simulink model "fixed_point_filter_converter"  (R2020a)
settings: Solver=FixedStepAuto  StartTime=0  StopTime=Inf  RelTol=1e-3
model workspace (MAT data in the model file):
  a = 0
settings Model: MinMaxOverflowLogging=MinMaxAndOverflow  FPTRunName=EmbeddedRun  FPTShortcutValueString='{{},{''BaselineRun_3'',1,1,1,''BaselineRun_3'','''',{},''M'',''D'',''''},{''EmbeddedRun'',1,1,1,''EmbeddedRun'','''',{},''M'','''',''''},{''BaselineRun'',1,1,1,''BaselineRun'','''',{},''M'',''D'',''''},{''BaselineRun_2'',1,1,1,''BaselineRun_2'','''',{},''M'',''D'',''''},{''EmbeddedRun_2'',1,1,1,''EmbeddedRun_2'','''',{},''M'','''',''''},{''BaselineRun_4'',1,1,1,''BaselineRun_4'','''',{},''M'',''D'',''''},{''BaselineRun_7'',1,1,1,''BaselineRun_7'','''',{},''M'',''D'',''''}}'  Creator=sbuccelli  LastModifiedBy=diflo
settings DataIOCC: SaveOutput=off  SaveTime=off
settings OptimizationCC: BlockReduction=off  ConditionallyExecuteInputs=off  DefaultParameterBehavior=Inlined
settings DebuggingCC: SignalRangeChecking=error  AlgebraicLoopMsg=error  SingleTaskRateTransMsg=error  IntegerOverflowMsg=none  ParameterDowncastMsg=none  ParameterOverflowMsg=none  ParameterPrecisionLossMsg=none  IntegerSaturationMsg=none
settings HardwareCC: ProdBitPerPointer=32  ProdBitPerSizeT=32  ProdBitPerPtrDiffT=32  ProdLargestAtomicFloat=None  ProdIntDivRoundTo=Undefined  ProdEndianess=Unspecified  ProdWordSize=32  ProdHWDeviceType=ASIC/FPGA->ASIC/FPGA  TargetBitPerPointer=64  TargetBitPerSizeT=64  TargetBitPerPtrDiffT=64  TargetLongLongMode=on  TargetIntDivRoundTo=Zero  TargetEndianess=LittleEndian  TargetWordSize=64  TargetHWDeviceType=Custom Processor->MATLAB Host Computer  ProdEqTarget=off

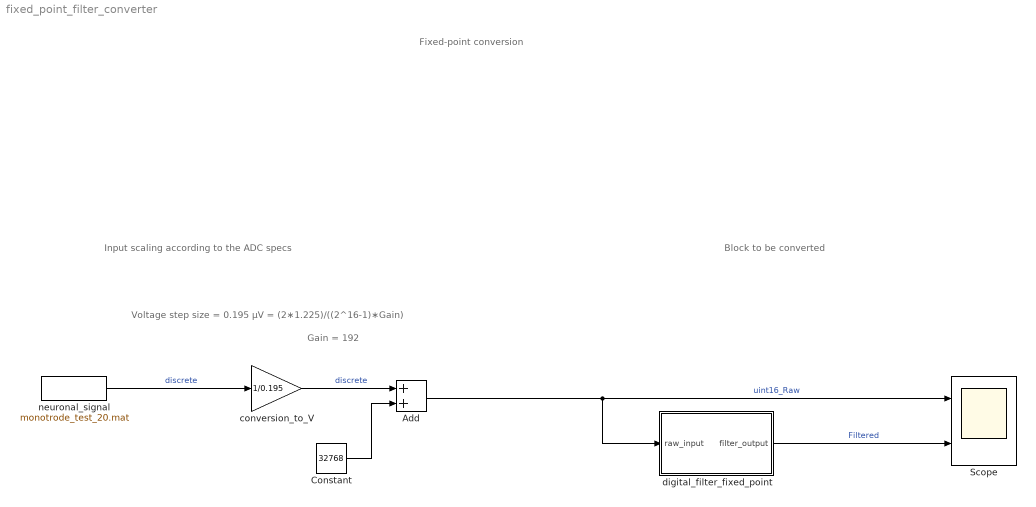
== system fixed_point_filter_converter ==
  note: Input scaling according to the ADC specs
  note: Gain = 192
  note: Voltage step size = 0.195 µV = (2∗1.225)/((2^16-1)∗Gain)
  note: Fixed-point conversion
  note: Block to be converted
  Add : Sum  OutDataTypeStr=uint16
  Constant : Constant  Value=32768  OutDataTypeStr=uint16  SampleTime=-1
  Scope : Scope  NumInputPorts=2
  conversion_to_V : Gain  Gain=1/0.195
  digital_filter_fixed_point : Subsystem
  neuronal_signal : FromFile  FileName=monotrode_test_20.mat  SampleTime=1/30000
  wires:
  neuronal_signal/1 -> conversion_to_V/1  "discrete"
  conversion_to_V/1 -> Add/1  "discrete"
  Constant/1 -> Add/2
  Add/1 -> digital_filter_fixed_point/1(raw_input), Scope/1  "uint16_Raw"
  digital_filter_fixed_point/1(filter_output) -> Scope/2  "Filtered"

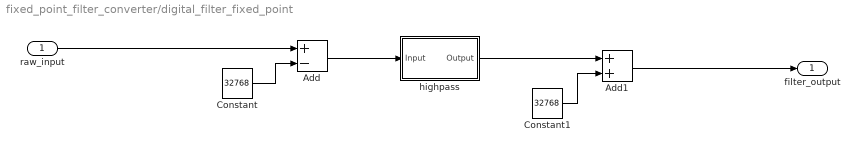
== system fixed_point_filter_converter/digital_filter_fixed_point ==
  raw_input : Inport  OutDataTypeStr=uint16  LockScale=on
  Add : Sum  Inputs=+-  AccumDataTypeStr=fixdt(1,32,14)  OutDataTypeStr=fixdt(1,32,15)  SaturateOnIntegerOverflow=on  LockScale=on
  Add1 : Sum  AccumDataTypeStr=fixdt(1,32,14)  OutDataTypeStr=uint16  SaturateOnIntegerOverflow=on  LockScale=on
  Constant : Constant  Value=32768  OutDataTypeStr=fixdt(0,16,0)  SampleTime=-1
  Constant1 : Constant  Value=32768  OutDataTypeStr=fixdt(0,16,0)  SampleTime=-1
  highpass : Subsystem  Tag=BlockMethodSubSystem
  filter_output : Outport  LockScale=on
  wires:
  Constant/1 -> Add/2
  Add/1 -> highpass/1(Input)
  Constant1/1 -> Add1/2
  highpass/1(Output) -> Add1/1
  raw_input/1 -> Add/1
  Add1/1 -> filter_output/1

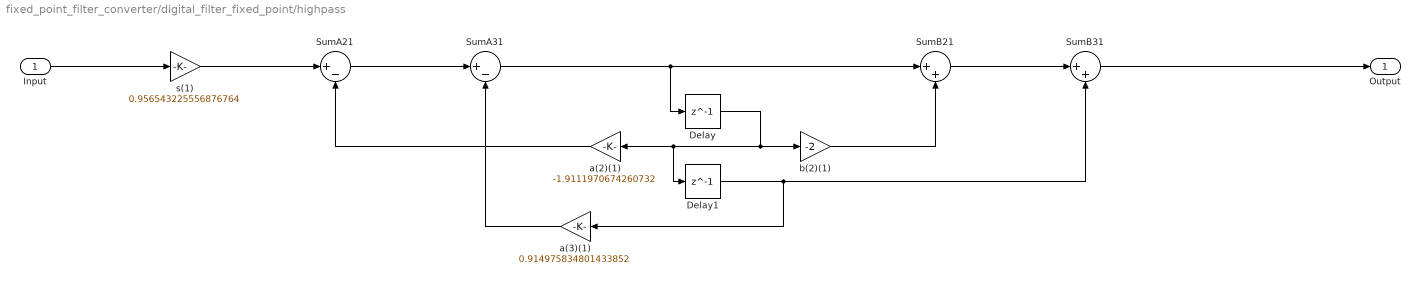
== system fixed_point_filter_converter/digital_filter_fixed_point/highpass ==
  Input : Inport  OutDataTypeStr=fixdt(1,32,15)
  Delay : Delay  DelayLength=1  InitialCondition=0
  Delay1 : Delay  DelayLength=1  InitialCondition=0
  SumA21 : Sum  Inputs=|+-  AccumDataTypeStr=fixdt(1,32,6)  OutDataTypeStr=fixdt(1,32,6)  RndMeth=Nearest  SaturateOnIntegerOverflow=on
  SumA31 : Sum  Inputs=|+-  AccumDataTypeStr=fixdt(1,32,6)  OutDataTypeStr=fixdt(1,32,7)  RndMeth=Nearest  SaturateOnIntegerOverflow=on
  SumB21 : Sum  Inputs=|++  AccumDataTypeStr=fixdt(1,32,6)  OutDataTypeStr=fixdt(1,32,7)  RndMeth=Nearest  SaturateOnIntegerOverflow=on
  SumB31 : Sum  Inputs=|++  AccumDataTypeStr=fixdt(1,32,7)  OutDataTypeStr=fixdt(1,32,15)  RndMeth=Nearest  SaturateOnIntegerOverflow=on
  a(2)(1) : Gain  Gain=-1.9111970674260732  ParamDataTypeStr=fixdt(1,32,30)  OutDataTypeStr=fixdt(1,32,6)  RndMeth=Nearest  SaturateOnIntegerOverflow=on
  a(3)(1) : Gain  Gain=0.914975834801433852  ParamDataTypeStr=fixdt(0,32,32)  OutDataTypeStr=fixdt(1,32,8)  RndMeth=Nearest  SaturateOnIntegerOverflow=on
  b(2)(1) : Gain  Gain=-2  ParamDataTypeStr=fixdt(1,32,30)  OutDataTypeStr=fixdt(1,32,6)  RndMeth=Nearest  SaturateOnIntegerOverflow=on
  s(1) : Gain  Gain=0.956543225556876764  ParamDataTypeStr=fixdt(0,32,32)  OutDataTypeStr=fixdt(1,32,16)  RndMeth=Nearest  SaturateOnIntegerOverflow=on
  Output : Outport  OutDataTypeStr=fixdt(1,32,15)
  wires:
  SumA21/1 -> SumA31/1
  SumB21/1 -> SumB31/1
  Input/1 -> s(1)/1
  a(2)(1)/1 -> SumA21/2
  s(1)/1 -> SumA21/1
  SumA31/1 -> Delay/1, SumB21/1
  b(2)(1)/1 -> SumB21/2
  SumB31/1 -> Output/1
  a(3)(1)/1 -> SumA31/2
  Delay/1 -> Delay1/1, a(2)(1)/1, b(2)(1)/1
  Delay1/1 -> a(3)(1)/1, SumB31/2
